simulink model "jarmuIranyitas"  (R2020b)
settings: Solver=VariableStepAuto  StartTime=0.0  StopTime=30  RelTol=1e-3
values from neighbouring files (symbols this model uses):
  b = 0.0011    [elorecsatoltszabalyzo.m]
  g = 9.81    [elorecsatoltszabalyzo.m]
  J = 0.1    [elorecsatoltszabalyzo.m]
  Kd_teta = 0.8    [elorecsatoltszabalyzo.m]
  Kd_y = 2*m*Eps*omega_n    (= 7.994)    [elorecsatoltszabalyzo.m]
  Kd_y_PID = (m/T)*(1+2*T*Eps*omega_n)    (= 17.994)    [elorecsatoltszabalyzo.m]
  Ki_y_PID = (m/T)*omega_n^2    (= 326.041)    [elorecsatoltszabalyzo.m]
  Kp_teta = 3.26    [elorecsatoltszabalyzo.m]
  Kp_y = m*omega_n^2    (= 32.6041)    [elorecsatoltszabalyzo.m]
  Kp_y_PID = (m/T)*(2*Eps*omega_n+T*omega_n^2)    (= 112.5441)    [elorecsatoltszabalyzo.m]
  l = 0.2    [elorecsatoltszabalyzo.m]
  m = 1    [elorecsatoltszabalyzo.m]
settings Model: Creator=Legion1  LastModifiedBy=Legion1

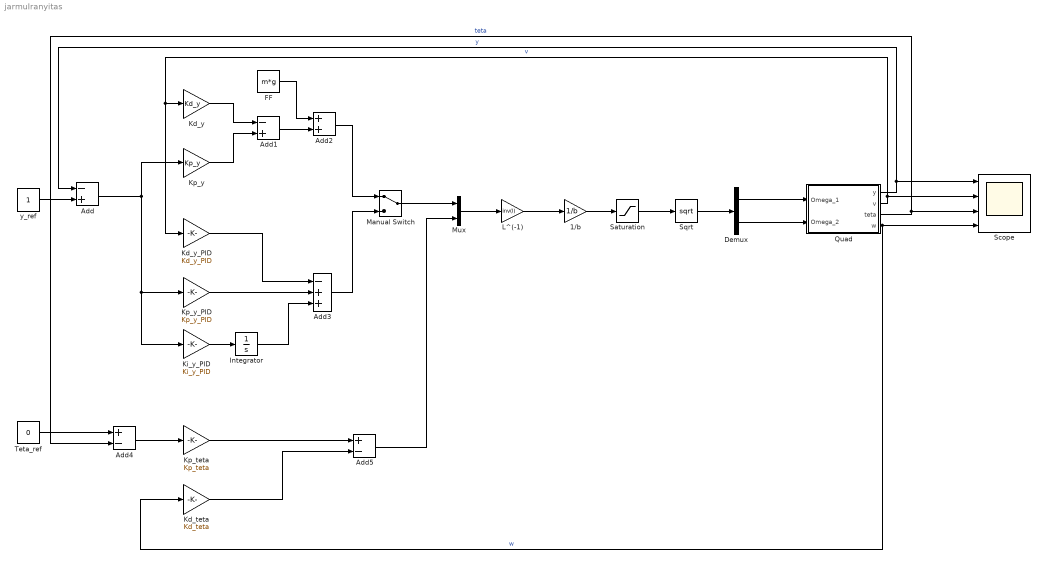
== system jarmuIranyitas ==
  1/b : Gain  Gain=1/b
  Add : Sum  Inputs=-+
  Add1 : Sum  Inputs=-+
  Add2 : Sum
  Add3 : Sum  Inputs=-++
  Add4 : Sum  Inputs=+-
  Add5 : Sum  Inputs=+-
  Demux : Demux  Outputs=2
  FF : Constant  Value=m*g
  Integrator : Integrator
  Kd_teta : Gain  Gain=Kd_teta
  Kd_y : Gain  Gain=Kd_y
  Kd_y_PID : Gain  Gain=Kd_y_PID
  Ki_y_PID : Gain  Gain=Ki_y_PID
  Kp_teta : Gain  Gain=Kp_teta
  Kp_y : Gain  Gain=Kp_y
  Kp_y_PID : Gain  Gain=Kp_y_PID
  L^(-1) : Gain  Gain=inv(l)
  Manual Switch : ManualSwitch
  Mux : Mux  Inputs=2
  Quad : Subsystem  mask{m=1, b=0.00110}
  Saturation : Saturate  UpperLimit=inf  LowerLimit=0
  Scope : Scope  NumInputPorts=4
  Sqrt : Sqrt  SaturateOnIntegerOverflow=on
  Teta_ref : Constant  Value=0
  y_ref : Constant
  wires:
  y_ref/1 -> Add/2
  Quad/1(y) -> Scope/1, Add/1  "y"
  Add/1 -> Kp_y/1, Kp_y_PID/1, Ki_y_PID/1
  Quad/2(v) -> Scope/2, Kd_y_PID/1, Kd_y/1  "v"
  Kd_y/1 -> Add1/1
  Kp_y/1 -> Add1/2
  Add1/1 -> Add2/2
  FF/1 -> Add2/1
  Kp_y_PID/1 -> Add3/2
  Kd_y_PID/1 -> Add3/1
  Ki_y_PID/1 -> Integrator/1
  Integrator/1 -> Add3/3
  Add2/1 -> Manual Switch/1
  Add3/1 -> Manual Switch/2
  Teta_ref/1 -> Add4/1
  Add4/1 -> Kp_teta/1
  Kp_teta/1 -> Add5/1
  Kd_teta/1 -> Add5/2
  Quad/3(teta) -> Scope/3, Add4/2  "teta"
  Quad/4(w) -> Kd_teta/1, Scope/4  "w"
  Manual Switch/1 -> Mux/1
  Add5/1 -> Mux/2
  Mux/1 -> L^(-1)/1
  L^(-1)/1 -> 1/b/1
  1/b/1 -> Saturation/1
  Saturation/1 -> Sqrt/1
  Sqrt/1 -> Demux/1
  Demux/1 -> Quad/1(Omega_1)
  Demux/2 -> Quad/2(Omega_2)

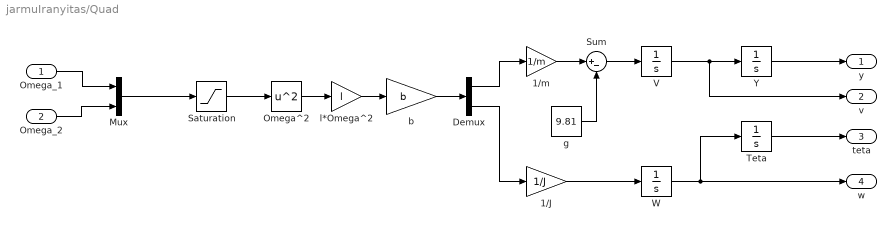
== system jarmuIranyitas/Quad ==
  Omega_1 : Inport
  Omega_2 : Inport  Port=2
  "1/J " : Gain  Gain=1/J
  1/m : Gain  Gain=1/m
  Demux : Demux  Outputs=2
  Mux : Mux  Inputs=2
  Omega^2 : Math  Operator=square  SignedPower=on  SaturateOnIntegerOverflow=on
  Saturation : Saturate  UpperLimit=inf  LowerLimit=0
  Sum : Sum  Inputs=|+-
  Teta : Integrator
  V : Integrator
  W : Integrator
  Y : Integrator
  b : Gain  Gain=b
  g : Constant  Value=9.81
  l*Omega^2 : Gain  Gain=l
  y : Outport  VectorParamsAs1DForOutWhenUnconnected=off
  v : Outport  Port=2  VectorParamsAs1DForOutWhenUnconnected=off
  teta : Outport  Port=3  VectorParamsAs1DForOutWhenUnconnected=off
  w : Outport  Port=4  VectorParamsAs1DForOutWhenUnconnected=off
  wires:
  Omega_2/1 -> Mux/2
  Omega_1/1 -> Mux/1
  Mux/1 -> Saturation/1
  Saturation/1 -> Omega^2/1
  Omega^2/1 -> l*Omega^2/1
  l*Omega^2/1 -> b/1
  b/1 -> Demux/1
  Demux/2 -> "1/J "/1
  Demux/1 -> 1/m/1
  "1/J "/1 -> W/1
  W/1 -> Teta/1, w/1
  V/1 -> v/1, Y/1
  Y/1 -> y/1
  Teta/1 -> teta/1
  1/m/1 -> Sum/1
  Sum/1 -> V/1
  g/1 -> Sum/2
